simulink model "Fuzzy_Block"  (R2023a)
settings: Solver=VariableStepAuto  StartTime=0.0  StopTime=20  RelTol=1e-3
libraries: fuzblock x1
settings Model: Creator=Alireza  LastModifiedBy=Alireza

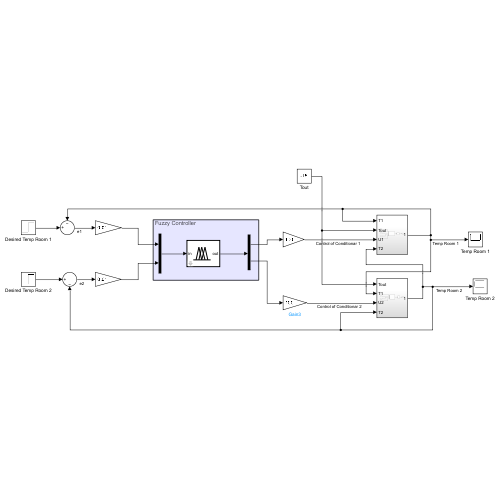
[thumbnail: Simulink's stored preview of the top-level diagram]
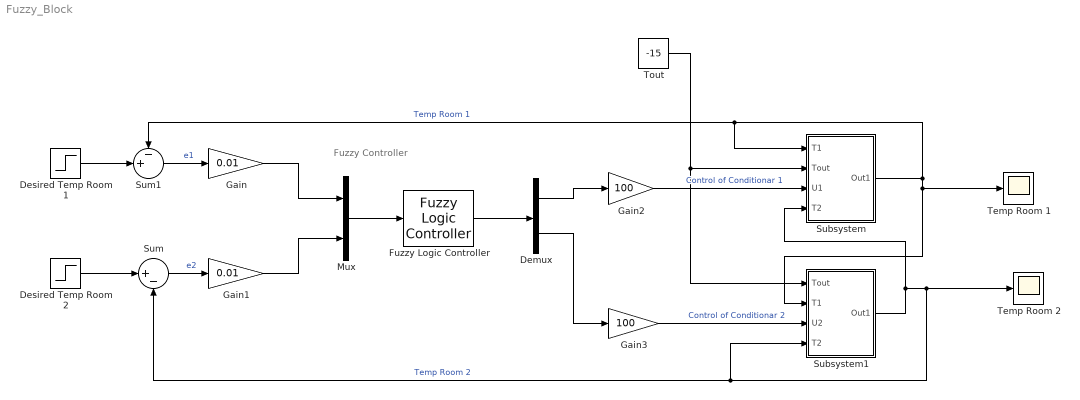
== system Fuzzy_Block ==
  note: Fuzzy Controller
  Demux : Demux  Outputs=2
  Desired Temp Room 1 : Step  Time=0  After=23  SampleTime=0
  Desired Temp Room 2 : Step  Time=0  After=37  SampleTime=0
  Fuzzy Logic Controller : fuzblock/Fuzzy Logic  Controller  FIS=FuzzyConditioner5  OutputSampleNumber=101  DataType=double  FuzzifiedInputs=off  RuleFiringStrengths=off  RuleOutputs=off  AggregatedOutputs=off  SimulateUsing=Interpreted execution  OutOfRangeInputValueMessage=warning  NoRuleFiredMessage=warning  EmptyOutputFuzzySetMessage=warning
  Gain : Gain  Gain=0.01
  Gain1 : Gain  Gain=0.01
  Gain2 : Gain  Gain=100
  Gain3 : Gain  Gain=100
  Mux : Mux  Inputs=2
  Subsystem : Subsystem
  Subsystem1 : Subsystem
  Sum : Sum  Inputs=|+-
  Sum1 : Sum  Inputs=-+|
  Temp Room 1 : Scope
  Temp Room 2 : Scope
  Tout : Constant  Value=-15
  wires:
  Desired Temp Room 1/1 -> Sum1/2
  Desired Temp Room 2/1 -> Sum/1
  Tout/1 -> Subsystem1/1(Tout), Subsystem/2(Tout)
  Sum/1 -> Gain1/1  "e2"
  Sum1/1 -> Gain/1  "e1"
  Demux/1 -> Gain2/1
  Demux/2 -> Gain3/1
  Gain1/1 -> Mux/2
  Fuzzy Logic Controller/1 -> Demux/1
  Gain/1 -> Mux/1
  Mux/1 -> Fuzzy Logic Controller/1
  Subsystem/1(Out1) -> Subsystem1/2(T1), Temp Room 1/1, Subsystem/1(T1), Sum1/1  "Temp Room 1"
  Gain2/1 -> Subsystem/3(U1)  "Control of Conditionar 1"
  Subsystem1/1(Out1) -> Subsystem/4(T2), Temp Room 2/1, Subsystem1/4(T2), Sum/2  "Temp Room 2"
  Gain3/1 -> Subsystem1/3(U2)  "Control of Conditionar 2"

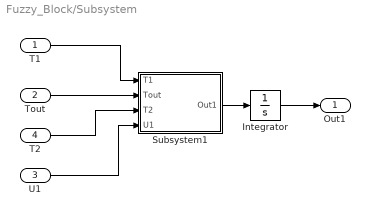
== system Fuzzy_Block/Subsystem ==
  T1 : Inport
  Tout : Inport  Port=2
  U1 : Inport  Port=3
  T2 : Inport  Port=4
  Integrator : Integrator
  Subsystem1 : Subsystem
  Out1 : Outport
  wires:
  T1/1 -> Subsystem1/1(T1)
  Subsystem1/1(Out1) -> Integrator/1
  Integrator/1 -> Out1/1
  T2/1 -> Subsystem1/3(T2)
  U1/1 -> Subsystem1/4(U1)
  Tout/1 -> Subsystem1/2(Tout)

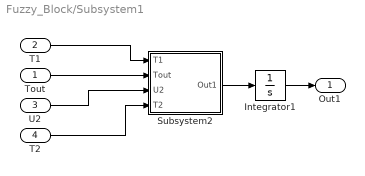
== system Fuzzy_Block/Subsystem1 ==
  Tout : Inport
  T1 : Inport  Port=2
  U2 : Inport  Port=3
  T2 : Inport  Port=4
  Integrator1 : Integrator
  Subsystem2 : Subsystem
  Out1 : Outport
  wires:
  Subsystem2/1(Out1) -> Integrator1/1
  U2/1 -> Subsystem2/3(U2)
  Integrator1/1 -> Out1/1
  T1/1 -> Subsystem2/1(T1)
  Tout/1 -> Subsystem2/2(Tout)
  T2/1 -> Subsystem2/4(T2)

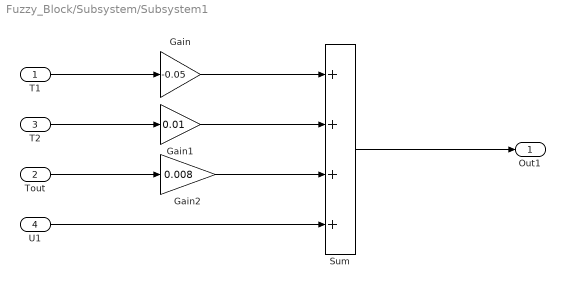
== system Fuzzy_Block/Subsystem/Subsystem1 ==
  T1 : Inport
  Tout : Inport  Port=2
  T2 : Inport  Port=3
  U1 : Inport  Port=4
  Gain : Gain  Gain=-0.05
  Gain1 : Gain  Gain=0.01
  Gain2 : Gain  Gain=0.008
  Sum : Sum  Inputs=++++
  Out1 : Outport
  wires:
  T1/1 -> Gain/1
  T2/1 -> Gain1/1
  Tout/1 -> Gain2/1
  U1/1 -> Sum/4
  Sum/1 -> Out1/1
  Gain/1 -> Sum/1
  Gain1/1 -> Sum/2
  Gain2/1 -> Sum/3

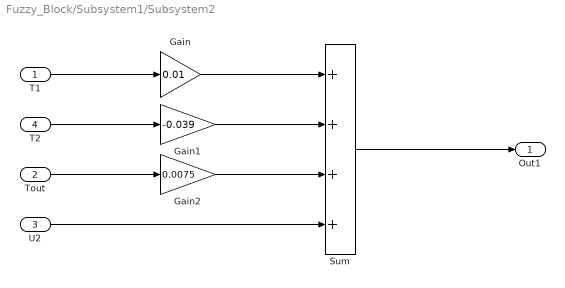
== system Fuzzy_Block/Subsystem1/Subsystem2 ==
  T1 : Inport
  Tout : Inport  Port=2
  U2 : Inport  Port=3
  T2 : Inport  Port=4
  Gain : Gain  Gain=0.01
  Gain1 : Gain  Gain=-0.039
  Gain2 : Gain  Gain=0.0075
  Sum : Sum  Inputs=++++
  Out1 : Outport
  wires:
  T1/1 -> Gain/1
  T2/1 -> Gain1/1
  Tout/1 -> Gain2/1
  U2/1 -> Sum/4
  Sum/1 -> Out1/1
  Gain/1 -> Sum/1
  Gain1/1 -> Sum/2
  Gain2/1 -> Sum/3
